simulink model "UKF_heli"  (R2017a)
settings: Solver=ode4  StartTime=0.0  StopTime=inf  FixedStep=0.1  RelTol=1e-3
InitFcn:
  | initialize_simulation
libraries: realtime_pacer_lib x1
settings Model: Creator=rosha  LastModifiedBy=rosha

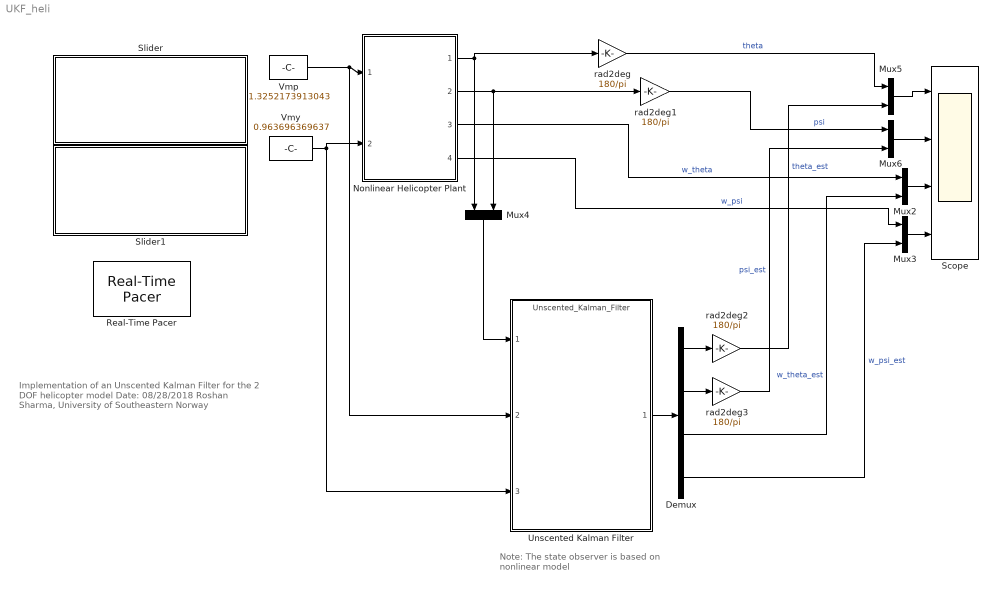
== system UKF_heli ==
  note: Implementation of an Unscented Kalman Filter
      | for the 2 DOF helicopter model
      | Date: 08/28/2018
      | Roshan Sharma, University of Southeastern Norway
  note: Note: The state observer is based on
      | nonlinear model
  Demux : Demux
  Mux{2..6} (5 alike) : Mux  Inputs=2
  Nonlinear Helicopter Plant : ModelReference  ModelNameDialog=Nonlinear_Helicopter_Plant  ModelReferenceVersion=1.161  CopyOfModelProtected=on
  Real-Time Pacer : realtime_pacer_lib/Real-Time Pacer  simTimePerRealTime=1
  Scope : Scope  NumInputPorts=4
  Slider : Subsystem  DialogController=hmiCreateDDGDialog  IsWebBlock=on  mask(MWDashboardBlock){webBlockId=65708a0b-0db9-4818-99ef-91d910a647f9, webBlockType=slider, ShowInLibBrowser=on, ShowInitialText=on, HMISrcModelName=UKF_heli}
      mask prompts: webBlockId "WebBlock Id"; webBlockType "WebBlock Type"; HMISrcModelName "Source Model"
      mask help: SimulinkHMI:dialogs:SliderDialogDesc
      mask Help: helpview([docroot '/mapfiles/simulink.map'], 'hmi_slider')
      mask Display:
      | if strcmp(get_param(bdroot(gcb),'BlockDiagramType'), 'library')
      |     image([(matlabroot) '/toolbox/simulink/hmi/icons/Slider.png']);
      | end
  Slider1 : Subsystem  DialogController=hmiCreateDDGDialog  IsWebBlock=on  mask(MWDashboardBlock){webBlockId=0ca4703d-b5a7-41b4-b347-6eb94f80e79f, webBlockType=slider, ShowInLibBrowser=on, ShowInitialText=on, HMISrcModelName=UKF_heli}
      mask prompts: webBlockId "WebBlock Id"; webBlockType "WebBlock Type"; HMISrcModelName "Source Model"
      mask help: SimulinkHMI:dialogs:SliderDialogDesc
      mask Help: helpview([docroot '/mapfiles/simulink.map'], 'hmi_slider')
      mask Display:
      | if strcmp(get_param(bdroot(gcb),'BlockDiagramType'), 'library')
      |     image([(matlabroot) '/toolbox/simulink/hmi/icons/Slider.png']);
      | end
  Unscented Kalman Filter : ModelReference  ModelNameDialog=Unscented_Kalman_Filter  ModelReferenceVersion=1.162  CopyOfModelProtected=on
  Vmp : Constant  Value=1.3252173913043
  Vmy : Constant  Value=0.963696369637
  rad2deg{,1..3} (4 alike) : Gain  Gain=180/pi
  wires:
  Vmp/1 -> Unscented Kalman Filter/2, Nonlinear Helicopter Plant/1
  Vmy/1 -> Unscented Kalman Filter/3, Nonlinear Helicopter Plant/2
  Nonlinear Helicopter Plant/1 -> rad2deg/1, Mux4/1
  rad2deg/1 -> Mux5/1  "theta"
  Nonlinear Helicopter Plant/2 -> rad2deg1/1, Mux4/2
  Nonlinear Helicopter Plant/3 -> Mux2/1  "w_theta"
  rad2deg1/1 -> Mux6/1  "psi"
  Mux2/1 -> Scope/3
  Mux3/1 -> Scope/4
  Nonlinear Helicopter Plant/4 -> Mux3/1  "w_psi"
  Mux4/1 -> Unscented Kalman Filter/1
  Unscented Kalman Filter/1 -> Demux/1
  Demux/1 -> rad2deg2/1
  Demux/2 -> rad2deg3/1
  Demux/3 -> Mux2/2  "w_theta_est"
  Demux/4 -> Mux3/2  "w_psi_est"
  rad2deg2/1 -> Mux5/2  "theta_est"
  rad2deg3/1 -> Mux6/2  "psi_est"
  Mux6/1 -> Scope/2
  Mux5/1 -> Scope/1

== system UKF_heli/Slider ==

== system UKF_heli/Slider1 ==
